simulink model "stage4b_pi_control"  (R2024a)
settings: Solver=FixedStepDiscrete  StartTime=0.0  StopTime=1800  FixedStep=10  RelTol=1e-3
settings Model: Creator=Peter  LastModifiedBy=Peter

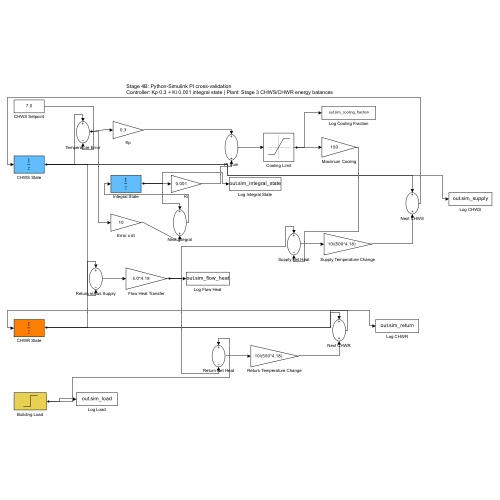
[thumbnail: Simulink's stored preview of the top-level diagram]
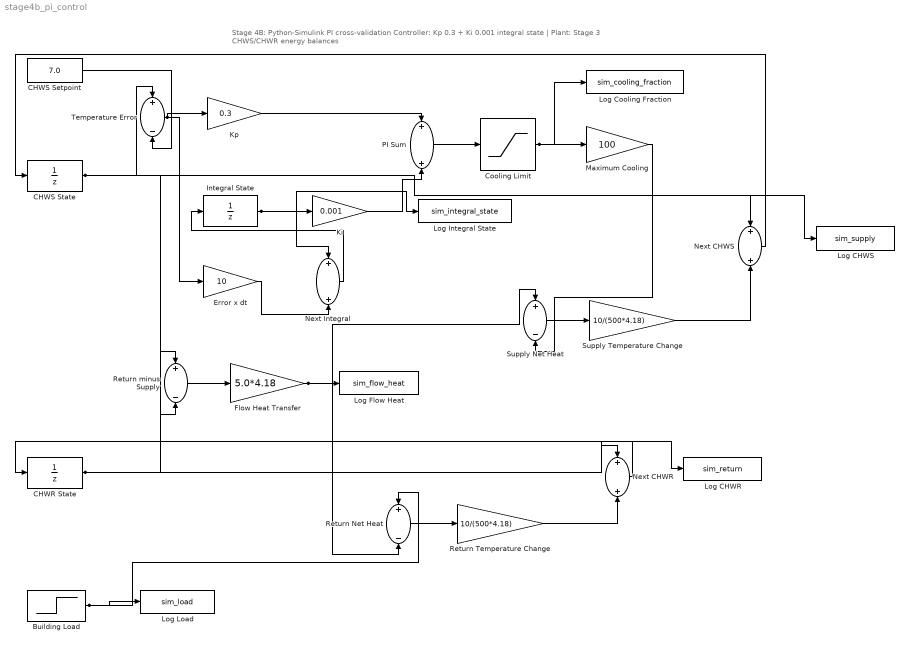
== system stage4b_pi_control ==
  note: Stage 4B: Python-Simulink PI cross-validation
      | Controller: Kp 0.3 + Ki 0.001 integral state | Plant: Stage 3 CHWS/CHWR energy balances
  Building Load : Step  Time=600  Before=30  After=50  SampleTime=10
  CHWR State : UnitDelay  InitialCondition=8.435406698564593  SampleTime=10  HasFrameUpgradeWarning=on
  CHWS Setpoint : Constant  Value=7.0
  CHWS State : UnitDelay  InitialCondition=7.0  SampleTime=10  HasFrameUpgradeWarning=on
  Cooling Limit : Saturate  UpperLimit=1  LowerLimit=0
  Error x dt : Gain  Gain=10
  Flow Heat Transfer : Gain  Gain=5.0*4.18
  Integral State : UnitDelay  InitialCondition=300  SampleTime=10  HasFrameUpgradeWarning=on
  Ki : Gain  Gain=0.001
  Kp : Gain  Gain=0.3
  Log CHWR : ToWorkspace  VariableName=sim_return  SaveFormat=Timeseries  SampleTime=-1
  Log CHWS : ToWorkspace  VariableName=sim_supply  SaveFormat=Timeseries  SampleTime=-1
  Log Cooling Fraction : ToWorkspace  VariableName=sim_cooling_fraction  SaveFormat=Timeseries  SampleTime=-1
  Log Flow Heat : ToWorkspace  VariableName=sim_flow_heat  SaveFormat=Timeseries  SampleTime=-1
  Log Integral State : ToWorkspace  VariableName=sim_integral_state  SaveFormat=Timeseries  SampleTime=-1
  Log Load : ToWorkspace  VariableName=sim_load  SaveFormat=Timeseries  SampleTime=-1
  Maximum Cooling : Gain  Gain=100
  Next CHWR : Sum
  Next CHWS : Sum
  Next Integral : Sum
  PI Sum : Sum
  Return Net Heat : Sum  Inputs=+-
  Return Temperature Change : Gain  Gain=10/(500*4.18)
  Return minus Supply : Sum  Inputs=+-
  Supply Net Heat : Sum  Inputs=+-
  Supply Temperature Change : Gain  Gain=10/(500*4.18)
  Temperature Error : Sum  Inputs=+-
  wires:
  CHWS State/1 -> Temperature Error/1, Return minus Supply/2, Next CHWS/1, Log CHWS/1
  CHWS Setpoint/1 -> Temperature Error/2
  Temperature Error/1 -> Kp/1, Error x dt/1
  Integral State/1 -> Ki/1, Next Integral/1, Log Integral State/1
  Error x dt/1 -> Next Integral/2
  Next Integral/1 -> Integral State/1
  Kp/1 -> PI Sum/1
  Ki/1 -> PI Sum/2
  PI Sum/1 -> Cooling Limit/1
  Cooling Limit/1 -> Maximum Cooling/1, Log Cooling Fraction/1
  CHWR State/1 -> Return minus Supply/1, Next CHWR/1, Log CHWR/1
  Return minus Supply/1 -> Flow Heat Transfer/1
  Flow Heat Transfer/1 -> Supply Net Heat/1, Return Net Heat/2, Log Flow Heat/1
  Maximum Cooling/1 -> Supply Net Heat/2
  Supply Net Heat/1 -> Supply Temperature Change/1
  Supply Temperature Change/1 -> Next CHWS/2
  Next CHWS/1 -> CHWS State/1
  Building Load/1 -> Return Net Heat/1, Log Load/1
  Return Net Heat/1 -> Return Temperature Change/1
  Return Temperature Change/1 -> Next CHWR/2
  Next CHWR/1 -> CHWR State/1
